simulink model "Compliance"  (R2020b)
settings: Solver=VariableStepAuto  StartTime=0.0  StopTime=4  RelTol=1e-3
values from neighbouring files (symbols this model uses):
  Kd = diag([2 10 30 1 1 1])    [params.m]
  Kp = diag([50 80 100 1 1 1])    [params.m]
  xd = Kinematics([t1,d2,d3], param)    [params.m]
settings Model: Creator=andre  LastModifiedBy=filippo

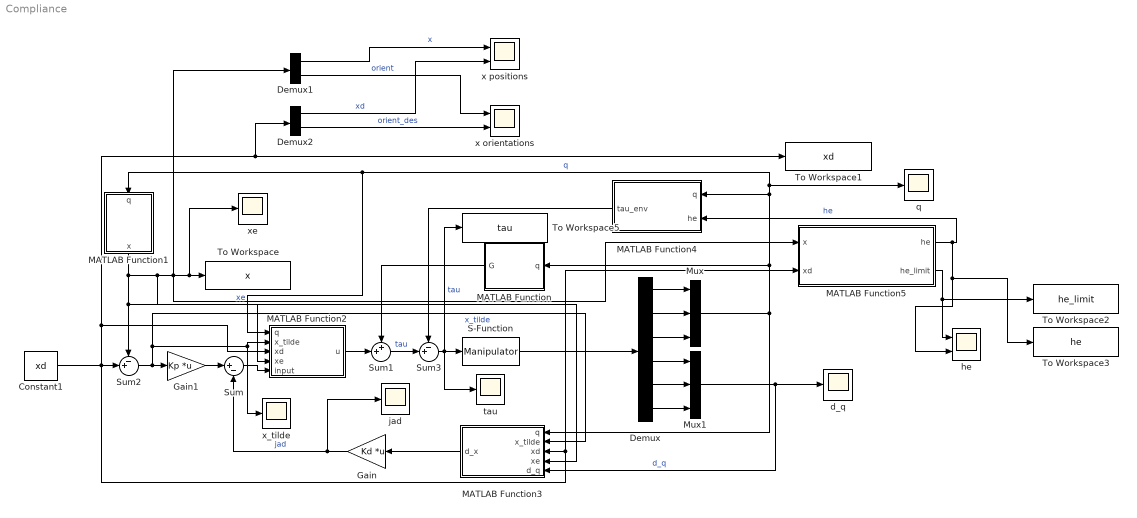
== system Compliance ==
  Constant1 : Constant  Value=xd
  Demux : Demux  Outputs=6
  Demux1 : Demux  Outputs=2
  Demux2 : Demux  Outputs=2
  Gain : Gain  Gain=Kd  Multiplication=Matrix(K*u)
  Gain1 : Gain  Gain=Kp  Multiplication=Matrix(K*u)
  MATLAB Function : MATLAB Function  TreatAsAtomicUnit=on
  MATLAB Function1 : MATLAB Function  TreatAsAtomicUnit=on
  MATLAB Function2 : MATLAB Function  TreatAsAtomicUnit=on
  MATLAB Function3 : MATLAB Function  TreatAsAtomicUnit=on
  MATLAB Function4 : MATLAB Function  TreatAsAtomicUnit=on
  MATLAB Function5 : MATLAB Function  TreatAsAtomicUnit=on
  Mux : Mux  Inputs=3
  Mux1 : Mux  Inputs=3
  S-Function : S-Function  FunctionName=Manipulator  Parameters=param  SFunctionDeploymentMode=off  EnableBusSupport=off
  Sum : Sum  Inputs=|+-
  Sum1 : Sum  Inputs=++|
  Sum2 : Sum  Inputs=-+|
  Sum3 : Sum  Inputs=-+|
  To Workspace : ToWorkspace  VariableName=x  SaveFormat=Timeseries  SampleTime=-1
  To Workspace1 : ToWorkspace  VariableName=xd  SaveFormat=Timeseries  SampleTime=-1
  To Workspace2 : ToWorkspace  VariableName=he_limit  SaveFormat=Timeseries  SampleTime=-1
  To Workspace3 : ToWorkspace  VariableName=he  SaveFormat=Timeseries  SampleTime=-1
  To Workspace5 : ToWorkspace  VariableName=tau  SaveFormat=Timeseries  SampleTime=-1
  d_q : Scope
  he : Scope  NumInputPorts=2
  jad : Scope
  q : Scope
  tau : Scope
  x orientations : Scope  NumInputPorts=2
  x positions : Scope  NumInputPorts=2
  x_tilde : Scope
  xe : Scope
  wires:
  Gain1/1 -> Sum/1
  S-Function/1 -> Demux/1
  Demux/3 -> Mux/3
  Demux/2 -> Mux/2
  Demux/1 -> Mux/1
  Demux/4 -> Mux1/1
  Demux/5 -> Mux1/2
  Demux/6 -> Mux1/3
  Mux/1 -> MATLAB Function3/1(q), MATLAB Function1/1(q), MATLAB Function2/1(q), q/1, MATLAB Function4/1(q), MATLAB Function/1(q)  "q"
  Gain/1 -> jad/1, Sum/2  "jad"
  Sum2/1 -> x_tilde/1, MATLAB Function2/2(x_tilde), MATLAB Function3/2(x_tilde), Gain1/1  "x_tilde"
  Mux1/1 -> MATLAB Function3/5(d_q), d_q/1  "d_q"
  Constant1/1 -> MATLAB Function5/2(xd), MATLAB Function3/3(xd), Sum2/2, MATLAB Function2/3(xd), Demux2/1, To Workspace1/1
  MATLAB Function1/1(x) -> MATLAB Function2/4(xe), Demux1/1, xe/1, To Workspace/1, MATLAB Function5/1(x), MATLAB Function3/4(xe), Sum2/1  "xe"
  MATLAB Function2/1(u) -> Sum1/2
  MATLAB Function3/1(d_x) -> Gain/1
  Demux1/1 -> x positions/1  "x"
  Demux2/1 -> x positions/2  "xd"
  Demux1/2 -> x orientations/1  "orient"
  Demux2/2 -> x orientations/2  "orient_des"
  Sum/1 -> MATLAB Function2/5(input)
  MATLAB Function5/1(he) -> To Workspace3/1, he/2, MATLAB Function4/2(he)  "he"
  Sum3/1 -> To Workspace5/1, tau/1, S-Function/1  "tau"
  MATLAB Function5/2(he_limit) -> To Workspace2/1, he/1
  Sum1/1 -> Sum3/2  "tau"
  MATLAB Function/1(G) -> Sum1/1
  MATLAB Function4/1(tau_env) -> Sum3/1

== matlab function Compliance/MATLAB Function1 ==
  data: q input; x output; param parameter
function x = Kin(q,param)
    x = Kinematics(q,param);
end

== matlab function Compliance/MATLAB Function ==
  data: q input; G output; param parameter
function G = Gravity(q, param)
   G = G_Lagrangian(q, param);
end

== matlab function Compliance/MATLAB Function2 ==
  data: q input; x_tilde input; xd input; xe input; input input; u output; param parameter
function u = JadT(q, x_tilde, xd,xe, input, param)
    Ja = getJad(q, x_tilde, xd, xe, param);
    u = Ja' * input;
end

== matlab function Compliance/MATLAB Function3 ==
  data: q input; x_tilde input; xd input; xe input; d_q input; d_x output; param parameter
function d_x = Jad(q, x_tilde, xd, xe, d_q, param)
    Ja = getJad(q, x_tilde, xd, xe, param);
    d_x = Ja * d_q;
end

== matlab function Compliance/MATLAB Function4 ==
  data: q input; he input; tau_env output; param parameter
function tau_env = JT(q, he, param)
    tau_env = Jacobian(q, param)' * he;
end

== matlab function Compliance/MATLAB Function5 ==
  data: x input; he output; xd input; param parameter; he_limit output
function [he, he_limit] = environment(x, xd, param)
    if x(param.axis) >= param.wall 

        % set up the rest position frame
        xr = zeros(6,1);
        xr(param.axis) = param.wall;

        xe = zeros(6,1);
        xe(param.axis) = x(param.axis);

        he = param.K * (xe - xr);
        dx_rd = zeros(6,1);
        dx_rd(param.axis) = xd(param.axis) - xr(param.axis);
        % At the limit
        he_limit =  param.K/(eye(6) + param.K / param.Kp) * dx_rd;
    else
        he = zeros(6,1);
        he_limit = zeros(6,1);
    end
end
